simulink model "testBranch"  (R2013b)
settings: Solver=ode45  StartTime=0.0  StopTime=10.0  RelTol=1e-3
settings Model: Creator=qiji  LastModifiedBy=qiji

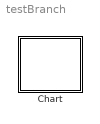
== system testBranch ==
  Chart : Stateflow chart  TreatAsAtomicUnit=on

== stateflow chart testBranch/Chart ==
